simulink model "sampleModel1730"  (R2023a)
settings: Solver=VariableStepAuto  StartTime=0.0  StopTime=10.0  RelTol=1e-3
libraries: hdlsllib x3, simulink x2
settings Model: Creator=user1  LastModifiedBy=user1

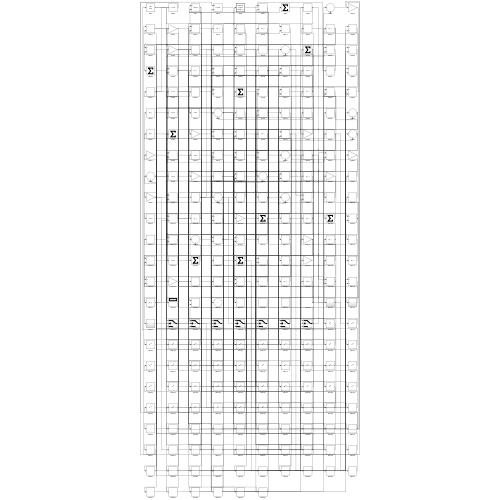
[thumbnail: Simulink's stored preview of the top-level diagram]
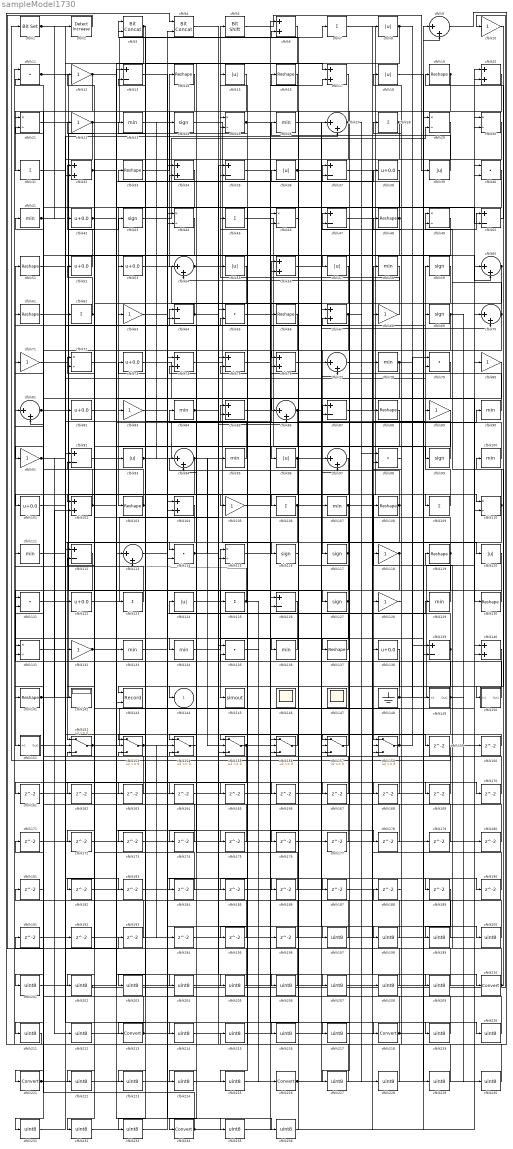
== system sampleModel1730 ==
  cfblk1 : simulink/Logic and Bit Operations/Bit Set  iBit=0
      settings: LibrarySourceBlock=|
      | hdlsllib/Logic and Bit
      | Operations/Bit Set
  cfblk{10,12,22,63,68,71,80,83,89,91,105,118,128,132} (14 alike) : Gain
  cfblk{23,26,41,58,78,84,90,95,100,107,111,129,133..134,136} (15 alike) : MinMax
  cfblk{38,42,52..53,73,82,101,122,138} (9 alike) : Bias  Bias=0.0  SaturateOnIntegerOverflow=off
  cfblk{6,17,20,32,34,56,67,74,76,85,102,104,140} (13 alike) : Sum
  cfblk{14,16,19,33,48,51,61,66,88,103,108,119,130,137,141} (15 alike) : Reshape
  cfblk{7,28,31,45,62,106,109,123,125} (9 alike) : Sum  Inputs=+
  cfblk{11,40,65,79,98,114,121,135} (8 alike) : DotProduct  OutDataTypeStr=Inherit: Inherit via internal rule
  cfblk{21,25,29..30,44,46,49,72,110,115,131} (11 alike) : Product  Inputs=*/  RndMeth=Zero  SaturateOnIntegerOverflow=on
  cfblk{13,35,37,47,50,64,75,87,92,112,126,139} (12 alike) : Sum  Inputs=+-
  cfblk{9,27,54,60,70,77,81,86,94,97,113} (11 alike) : Sum  Inputs=|++
  cfblk{24,43,59,69,99,116..117,127} (8 alike) : Signum
  cfblk{8,15,18,36,39,55,57,93,96,120,124} (11 alike) : Abs  SaturateOnIntegerOverflow=off
  cfblk142 : Display
  cfblk143 : Record  FileSettingsInternal="{\"entries\":[{\"content\":{\"excelSettings\":{\"content\":{},\"type\":\"Streamout.ExcelSettings\"}},\"type\":\"Streamout.FileSettingStorage\",\"uuid\":\"\"}],\"packageUris\":[\"http:\\/\\/schema.mathworks.com\\/mf0\\/streamout_blocks\\/R2020a\"],\"version\":\"1.0\"}"  Layout=[1 1]  SignalsInternal="{\"entries\":[{\"content\":{\"signals\":[{\"content\":{\"blockPath\":[],\"dimensions\":[1],\"domain\":\"\",\"lineColor\":\"#a2142f\",\"plots\":[1],\"port\":1,\"signalID\":3450,\"signalName\":\"XY Graph:1\"},\"type\":\"RecordBlkView.Signal\",\"uuid\":\"\"},{\"content\":{\"blockPath\":[],\"dimensions\":[1],\"domain\":\"\",\"lineColor\":\"#139fff\",\"plots\":[1],\"port\":2,\"signalID\":3453,\"signalName\":\"XY Graph:2\"},\"type\":\"RecordBlkView.Signal\",\"uuid\":\"\"}]},\"type\":\"RecordBlkView.InputSignals\",\"uuid\":\"\"}],\"packageUris\":[\"http:\\/\\/schema.mathworks.com\\/mf0\\/streamout_blocks\\/R2020a\"],\"version\":\"1.0\"}"  VisualizationBindings="{\"xyplotplugin\":{\"info\":[{\"series\":[{\"bindingParametersList\":[{\"parameter\":\"X-Axis\",\"signalID\":3450,\"signalName\":\"XY Graph:1\"},{\"parameter\":\"Y-Axis\",\"signalID\":3453,\"signalName\":\"XY Graph:2\"}],\"seriesID\":18890}],\"subplotID\":1}]}}"  CompatibilityTag=XY  st=-1
  cfblk145 : ToWorkspace  VariableName=simout  SaveFormat=Timeseries  SampleTime=-1
  cfblk146 : Scope
      settings: Floating=on
  cfblk147 : Scope
      settings: Floating=on
  cfblk148 : Ground
  cfblk149 : Subsystem
      settings: LibrarySourceBlock=|
      | hdlsllib/Ports &
      | Subsystems/Subsystem
  cfblk150 : Subsystem
      settings: LibrarySourceBlock=|
      | hdlsllib/Ports &
      | Subsystems/Subsystem
  cfblk151 : Subsystem
      settings: LibrarySourceBlock=|
      | hdlsllib/Ports &
      | Subsystems/Subsystem
  cfblk{152..158} (7 alike) : Switch  SaturateOnIntegerOverflow=off  InputSameDT=off
  cfblk{159..196} (38 alike) : Delay  SampleTime=1
  cfblk{197..209,211..212,214..217,219..220,222..225,227..233,235..236} (34 alike) : DataTypeConversion  OutDataTypeStr=uint8  SaturateOnIntegerOverflow=off  RndMeth=Floor
  cfblk2 : simulink/Logic and Bit Operations/Detect Increase  vinit=0.0  OutDataTypeStr=boolean
      settings: LibrarySourceBlock=|
      | hdlsllib/Logic and Bit
      | Operations/Detect
      | Increase
  cfblk{210,213,218,221,226,234} (6 alike) : DataTypeConversion  SaturateOnIntegerOverflow=off  RndMeth=Floor
  cfblk3 : hdlsllib/Logic and Bit Operations/Bit Concat  numInputs=2
  cfblk4 : hdlsllib/Logic and Bit Operations/Bit Concat  numInputs=2
  cfblk5 : hdlsllib/Logic and Bit Operations/Bit Shift  mode=Shift Left Logical  N=0
  cfblk144 : Outport  VectorParamsAs1DForOutWhenUnconnected=off
  wires:
  cfblk150/1(Out1) -> cfblk51/1
  cfblk153/1 -> cfblk129/1, cfblk194/1
  cfblk109/1 -> cfblk59/1
  cfblk68/1 -> cfblk5/1
  cfblk34/1 -> cfblk103/1
  cfblk141/1 -> cfblk25/1, cfblk102/2
  cfblk121/1 -> cfblk43/1
  cfblk21/1 -> cfblk127/1
  cfblk67/1 -> cfblk201/1, cfblk228/1
  cfblk3/1 -> cfblk53/1, cfblk153/2
  cfblk33/1 -> cfblk14/1
  cfblk112/1 -> cfblk151/1(In1)
  cfblk62/1 -> cfblk52/1, cfblk102/1
  cfblk119/1 -> cfblk64/1, cfblk185/1
  cfblk24/1 -> cfblk116/1
  cfblk88/1 -> cfblk114/1
  cfblk50/1 -> cfblk19/1
  cfblk132/1 -> cfblk90/1, cfblk157/3
  cfblk71/1 -> cfblk109/1
  cfblk45/1 -> cfblk99/1
  cfblk4/1 -> cfblk210/1
  cfblk46/1 -> cfblk136/1
  cfblk11/1 -> cfblk93/1, cfblk114/2
  cfblk80/1 -> cfblk221/1
  cfblk136/1 -> cfblk134/1
  cfblk104/1 -> cfblk152/1
  cfblk100/1 -> cfblk84/1
  cfblk15/1 -> cfblk31/1
  cfblk42/1 -> cfblk37/1, cfblk96/1
  cfblk125/1 -> cfblk113/2, cfblk196/1
  cfblk55/1 -> cfblk64/2
  cfblk6/1 -> cfblk234/1
  cfblk99/1 -> cfblk3/1
  cfblk103/1 -> cfblk33/1, cfblk42/1
  cfblk59/1 -> cfblk144/1
  cfblk5/1 -> cfblk39/1
  cfblk28/1 -> cfblk154/1, cfblk217/1
  cfblk70/1 -> cfblk117/1, cfblk153/1, cfblk49/2
  cfblk107/1 -> cfblk122/1, cfblk89/1
  cfblk73/1 -> cfblk130/1
  cfblk123/1 -> cfblk111/1
  cfblk69/1 -> cfblk126/2, cfblk155/3, cfblk160/1
  cfblk134/1 -> cfblk115/1
  cfblk40/1 -> cfblk105/1
  cfblk65/1 -> cfblk218/1
  cfblk106/1 -> cfblk70/2, cfblk172/1, cfblk173/1
  cfblk93/1 -> cfblk56/1, cfblk88/1, cfblk24/1
  cfblk74/1 -> cfblk158/1
  cfblk131/1 -> cfblk82/1
  cfblk54/1 -> cfblk86/2, cfblk167/1, cfblk206/1
  cfblk126/1 -> cfblk131/1
  cfblk1/1 -> cfblk112/1, cfblk17/1
  cfblk20/1 -> cfblk104/2
  cfblk122/1 -> cfblk55/1
  cfblk84/1 -> cfblk186/1, cfblk187/1
  cfblk36/1 -> cfblk76/1, cfblk198/1
  cfblk91/1 -> cfblk62/1, cfblk212/1
  cfblk85/1 -> cfblk46/2
  cfblk113/1 -> cfblk36/1
  cfblk29/1 -> cfblk132/1
  cfblk7/1 -> cfblk110/1
  cfblk129/1 -> cfblk58/1
  cfblk110/1 -> cfblk49/1, cfblk164/1
  cfblk8/1 -> cfblk149/1(In1), cfblk203/1
  cfblk19/1 -> cfblk107/1, cfblk86/1
  cfblk22/1 -> cfblk7/1, cfblk60/2, cfblk50/2, cfblk32/2
  cfblk118/1 -> cfblk137/1, cfblk232/1
  cfblk60/1 -> cfblk156/2, cfblk222/1
  cfblk13/1 -> cfblk110/2
  cfblk32/1 -> cfblk87/2, cfblk205/1
  cfblk39/1 -> cfblk26/1
  cfblk82/1 -> cfblk113/1
  cfblk26/1 -> cfblk120/1
  cfblk41/1 -> cfblk2/1, cfblk214/1
  cfblk108/1 -> cfblk94/1, cfblk195/1
  cfblk139/1 -> cfblk15/1, cfblk184/1
  cfblk151/1(Out1) -> cfblk85/1
  cfblk156/1 -> cfblk155/1
  cfblk76/1 -> cfblk50/1
  cfblk12/1 -> cfblk91/1, cfblk175/1
  cfblk81/1 -> cfblk27/2, cfblk21/2, cfblk79/2
  cfblk111/1 -> cfblk69/1
  cfblk89/1 -> cfblk143/1
  cfblk10/1 -> cfblk150/1(In1)
  cfblk98/1 -> cfblk28/1
  cfblk17/1 -> cfblk83/1
  cfblk53/1 -> cfblk97/2
  cfblk155/1 -> cfblk17/2, cfblk189/1, cfblk211/1
  cfblk116/1 -> cfblk56/2
  cfblk124/1 -> cfblk145/1
  cfblk38/1 -> cfblk121/1
  cfblk52/1 -> cfblk32/1
  cfblk137/1 -> cfblk124/1
  cfblk30/1 -> cfblk106/1
  cfblk130/1 -> cfblk125/1
  cfblk94/1 -> cfblk141/1, cfblk155/2
  cfblk25/1 -> cfblk47/2, cfblk219/1
  cfblk90/1 -> cfblk61/1
  cfblk78/1 -> cfblk143/2, cfblk139/1
  cfblk51/1 -> cfblk57/1
  cfblk96/1 -> cfblk67/1, cfblk76/2, cfblk233/1
  cfblk127/1 -> cfblk16/1, cfblk162/1
  cfblk138/1 -> cfblk213/1
  cfblk114/1 -> cfblk95/1, cfblk178/1
  cfblk128/1 -> cfblk48/1
  cfblk148/1 -> cfblk78/1, cfblk70/1, cfblk72/2
  cfblk64/1 -> cfblk63/1, cfblk139/2
  cfblk95/1 -> cfblk23/1
  cfblk158/1 -> cfblk22/1, cfblk79/1
  cfblk115/1 -> cfblk38/1
  cfblk102/1 -> cfblk87/1, cfblk41/1, cfblk236/1
  cfblk152/1 -> cfblk13/1, cfblk30/2
  cfblk87/1 -> cfblk8/1
  cfblk14/1 -> cfblk54/1
  cfblk48/1 -> cfblk101/1, cfblk34/2, cfblk13/2
  cfblk135/1 -> cfblk226/1
  cfblk72/1 -> cfblk123/1
  cfblk27/1 -> cfblk21/1, cfblk98/1, cfblk163/1
  cfblk47/1 -> cfblk68/1
  cfblk117/1 -> cfblk12/1, cfblk174/1
  cfblk63/1 -> cfblk37/2
  cfblk86/1 -> cfblk142/1, cfblk168/1
  cfblk43/1 -> cfblk29/2
  cfblk58/1 -> cfblk54/2
  cfblk154/1 -> cfblk74/2
  cfblk149/1(Out1) -> cfblk47/1, cfblk156/3, cfblk230/1
  cfblk157/1 -> cfblk72/1
  cfblk61/1 -> cfblk159/1
  cfblk159/1 -> cfblk1/1
  cfblk160/1 -> cfblk157/1
  cfblk16/1 -> cfblk161/1
  cfblk161/1 -> cfblk97/1
  cfblk163/1 -> cfblk131/2
  cfblk164/1 -> cfblk27/1
  cfblk49/1 -> cfblk165/1
  cfblk101/1 -> cfblk166/1
  cfblk166/1 -> cfblk29/1
  cfblk167/1 -> cfblk25/2
  cfblk168/1 -> cfblk34/1
  cfblk105/1 -> cfblk169/1
  cfblk169/1 -> cfblk85/2
  cfblk37/1 -> cfblk170/1
  cfblk170/1 -> cfblk81/2
  cfblk171/1 -> cfblk46/1
  cfblk172/1 -> cfblk154/2
  cfblk173/1 -> cfblk115/2
  cfblk174/1 -> cfblk121/2
  cfblk175/1 -> cfblk94/2
  cfblk57/1 -> cfblk176/1
  cfblk176/1 -> cfblk20/1
  cfblk56/1 -> cfblk177/1
  cfblk177/1 -> cfblk74/1
  cfblk178/1 -> cfblk67/2
  cfblk179/1 -> cfblk152/2
  cfblk180/1 -> cfblk157/2
  cfblk181/1 -> cfblk11/2
  cfblk120/1 -> cfblk182/1
  cfblk182/1 -> cfblk126/1
  cfblk31/1 -> cfblk183/1
  cfblk183/1 -> cfblk156/1
  cfblk184/1 -> cfblk152/3
  cfblk185/1 -> cfblk158/3
  cfblk186/1 -> cfblk154/3
  cfblk188/1 -> cfblk98/2
  cfblk83/1 -> cfblk190/1
  cfblk190/1 -> cfblk158/2
  cfblk191/1 -> cfblk30/1
  cfblk192/1 -> cfblk104/1
  cfblk2/1 -> cfblk193/1
  cfblk193/1 -> cfblk112/2
  cfblk194/1 -> cfblk60/1
  cfblk195/1 -> cfblk3/2
  cfblk196/1 -> cfblk73/1
  cfblk35/1 -> cfblk197/1
  cfblk197/1 -> cfblk45/1
  cfblk198/1 -> cfblk35/1
  cfblk189/1 -> cfblk199/1
  cfblk199/1 -> cfblk35/2
  cfblk133/1 -> cfblk200/1
  cfblk200/1 -> cfblk171/1
  cfblk201/1 -> cfblk133/1
  cfblk66/1 -> cfblk202/1
  cfblk202/1 -> cfblk10/1
  cfblk203/1 -> cfblk66/1
  cfblk92/1 -> cfblk204/1
  cfblk204/1 -> cfblk40/2
  cfblk205/1 -> cfblk92/1
  cfblk206/1 -> cfblk92/2
  cfblk75/1 -> cfblk207/1
  cfblk207/1 -> cfblk40/1
  cfblk208/1 -> cfblk75/1
  cfblk77/1 -> cfblk209/1
  cfblk209/1 -> cfblk75/2
  cfblk210/1 -> cfblk188/1, cfblk100/1, cfblk119/1
  cfblk211/1 -> cfblk4/1
  cfblk212/1 -> cfblk4/2
  cfblk213/1 -> cfblk191/1, cfblk118/1
  cfblk214/1 -> cfblk138/1
  cfblk9/1 -> cfblk215/1
  cfblk215/1 -> cfblk77/1
  cfblk79/1 -> cfblk216/1
  cfblk216/1 -> cfblk9/1
  cfblk217/1 -> cfblk9/2
  cfblk218/1 -> cfblk153/3, cfblk81/1
  cfblk219/1 -> cfblk65/1
  cfblk162/1 -> cfblk220/1
  cfblk220/1 -> cfblk65/2
  cfblk221/1 -> cfblk128/1, cfblk71/1
  cfblk222/1 -> cfblk80/1
  cfblk140/1 -> cfblk223/1
  cfblk223/1 -> cfblk108/1
  cfblk97/1 -> cfblk224/1
  cfblk224/1 -> cfblk140/1
  cfblk165/1 -> cfblk225/1
  cfblk225/1 -> cfblk140/2
  cfblk226/1 -> cfblk20/2, cfblk77/2
  cfblk187/1 -> cfblk227/1
  cfblk227/1 -> cfblk135/1
  cfblk228/1 -> cfblk135/2
  cfblk18/1 -> cfblk229/1
  cfblk229/1 -> cfblk11/1
  cfblk230/1 -> cfblk18/1
  cfblk44/1 -> cfblk231/1
  cfblk231/1 -> cfblk192/1
  cfblk232/1 -> cfblk44/1
  cfblk233/1 -> cfblk44/2
  cfblk234/1 -> cfblk208/1, cfblk181/1, cfblk180/1, cfblk179/1
  cfblk23/1 -> cfblk235/1
  cfblk235/1 -> cfblk6/1
  cfblk236/1 -> cfblk6/2

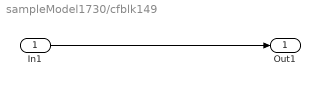
== system sampleModel1730/cfblk149 ==
  In1 : Inport
  Out1 : Outport
  wires:
  In1/1 -> Out1/1

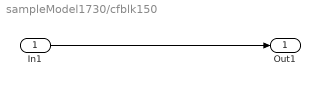
== system sampleModel1730/cfblk150 ==
  In1 : Inport
  Out1 : Outport
  wires:
  In1/1 -> Out1/1

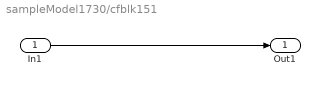
== system sampleModel1730/cfblk151 ==
  In1 : Inport
  Out1 : Outport
  wires:
  In1/1 -> Out1/1
